simulink model "Model_Following_Destrete"  (Simulink 8.5)
settings: Solver=ode45  StartTime=0.0  StopTime=5  RelTol=1e-3
values from neighbouring files (symbols this model uses):
  A = []    [AMB_5DOF_Destrete.m]
  B = []    [AMB_5DOF_Destrete.m]
  C = []    [AMB_5DOF_Destrete.m]
  C_ok = [-0.460327722928 -0.895193320177 -0.499481696109 -0.835473132173 -0.52391497842 -0.128357093475 -0.642598022326 -0.00646060119268 -0.752510607312 0.198829034268 -0.111610486964 0.0295345798937 ... (50 elements, 5x10)]    [okdata.mat]
  Cd = 0    [AMB_5DOF_Destrete.m]
  Cu_star = inv(Rd_wave)*(H'*inv((G-H*Kd)'-eye(nr))*Kd'+eye(mr))*Rd    [AMB_5DOF_Destrete.m]
  D = zeros(size(C,1),size(B,2))    [AMB_5DOF_Destrete.m]
  Ed = inv(Rd_wave)*(D'+H'*inv(eye(nr)-(G-H*Kd)')*(C-D*Kd)')*Qd    [AMB_5DOF_Destrete.m]
  F_ok = [0.353674763635 -0.0788531754208 0.0140079710216 -0.010986655228 0.000143400444828 -0.000393322361311 8.11625508598e-05 0.00568532225361 0.000196004583795 0.000136636780908 0.13443303816 0.417641667468 ... (50 elements, 10x5)]    [okdata.mat]
  G = G_ok    [AMB_5DOF_Destrete.m]
  H = H_ok    [AMB_5DOF_Destrete.m]
  Ts = 0.01    [AMB_5DOF_Destrete.m]
  ud_star = [0 0 0 0 0]'    [AMB_5DOF_Destrete.m]
undefined symbols (not defined in the file or in its folder): Kd, x
settings Model: Creator=koni  LastModifiedBy=123
settings DebuggingCC: SolverPrmCheckMsg=warning  FcnCallInpInsideContextMsg=UseLocalSettings

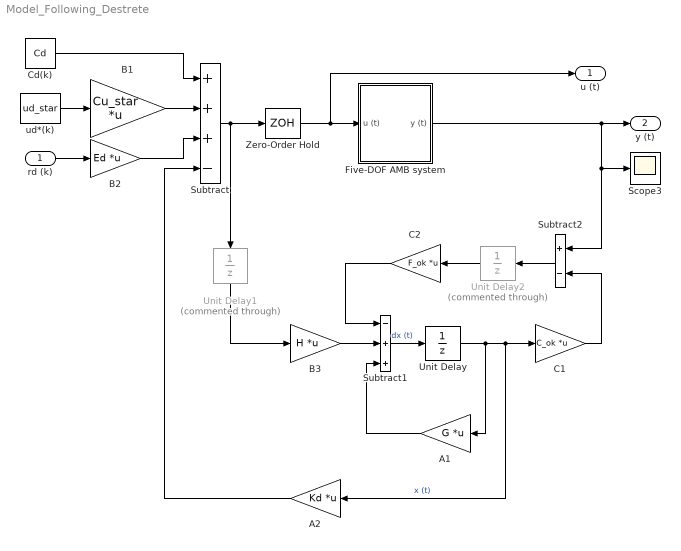
== system Model_Following_Destrete ==
  rd (k) : Inport  PortDimensions=pr
  " Five-DOF AMB system" : Subsystem
  A1 : Gain  Gain=G  Multiplication=Matrix(K*u)
  A2 : Gain  Gain=Kd  Multiplication=Matrix(K*u)
  B1 : Gain  Gain=Cu_star  Multiplication=Matrix(K*u)
  B2 : Gain  Gain=Ed  Multiplication=Matrix(K*u)
  B3 : Gain  Gain=H  Multiplication=Matrix(K*u)
  C1 : Gain  Gain=C_ok  Multiplication=Matrix(K*u)
  C2 : Gain  Gain=F_ok  Multiplication=Matrix(K*u)
  Cd(k) : Constant  Value=Cd
  Scope3 : Scope
      settings: TimeRange=0.05
  Subtract : Sum  Inputs=+++-
  Subtract1 : Sum  Inputs=-++
  Subtract2 : Sum  Inputs=+-
  Unit Delay : UnitDelay  SampleTime=Ts
  Unit Delay1 : UnitDelay  Commented=through  SampleTime=-1
  Unit Delay2 : UnitDelay  Commented=through  SampleTime=-1
  Zero-Order Hold : ZeroOrderHold  SampleTime=Ts
  ud*(k) : Constant  Value=ud_star
  u (t) : Outport  PortDimensions=mr
  y (t) : Outport  Port=2  PortDimensions=pr
  wires:
  " Five-DOF AMB system"/1(y (t)) -> Scope3/1, Subtract2/1, y (t)/1
  B2/1 -> Subtract/3
  rd (k)/1 -> B2/1
  ud*(k)/1 -> B1/1
  B1/1 -> Subtract/2
  Cd(k)/1 -> Subtract/1
  Zero-Order Hold/1 -> " Five-DOF AMB system"/1(u (t)), u (t)/1
  C1/1 -> Subtract2/2
  A1/1 -> Subtract1/3
  B3/1 -> Subtract1/2
  C2/1 -> Subtract1/1
  A2/1 -> Subtract/4
  Subtract1/1 -> Unit Delay/1  "dx (t)"
  Subtract2/1 -> Unit Delay2/1
  Subtract/1 -> Unit Delay1/1, Zero-Order Hold/1
  Unit Delay1/1 -> B3/1
  Unit Delay/1 -> A2/1, C1/1, A1/1  "x (t)"
  Unit Delay2/1 -> C2/1

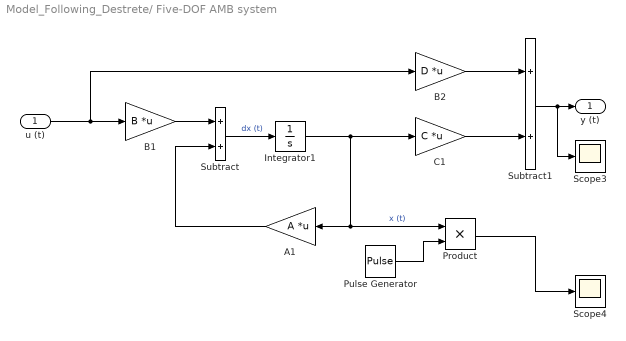
== system Model_Following_Destrete/ Five-DOF AMB system ==
  u (t) : Inport  PortDimensions=mr
  A1 : Gain  Gain=A  Multiplication=Matrix(K*u)
  B1 : Gain  Gain=B  Multiplication=Matrix(K*u)
  B2 : Gain  Gain=D  Multiplication=Matrix(K*u)
  C1 : Gain  Gain=C  Multiplication=Matrix(K*u)
  Integrator1 : Integrator  InitialCondition=x(:,1)
  Product : Product
  Pulse Generator : DiscretePulseGenerator  PulseType=Time based  Period=Ts
  Scope3 : Scope
      settings: TimeRange=0.05  SaveName=ScopeData2
  Scope4 : Scope
      settings: TimeRange=0.04999  YMin=-0.001  YMax=0.006  SaveName=ScopeData3
  Subtract : Sum
  Subtract1 : Sum
  y (t) : Outport  PortDimensions=pr
  wires:
  Subtract/1 -> Integrator1/1  "dx (t)"
  Integrator1/1 -> C1/1, A1/1, Product/1  "x (t)"
  u (t)/1 -> B1/1, B2/1
  B1/1 -> Subtract/1
  A1/1 -> Subtract/2
  Subtract1/1 -> Scope3/1, y (t)/1
  C1/1 -> Subtract1/2
  B2/1 -> Subtract1/1
  Product/1 -> Scope4/1
  Pulse Generator/1 -> Product/2
